simulink model "Benchmark2021ControllerNew"  (R2018a)
settings: Solver=ode1  StartTime=0  StopTime=t_end  FixedStep=simTs  RelTol=1e-3
values from neighbouring files (symbols this model uses):
  Horizon_Lowlayer = T_PreDomn-T_Apply    [Initial_Lower.m]
  Initial_headway = Sensor_FOL_dDist(2)    [Initial_main.m]
  Initial_MG1_spd = 0    [Initial_Lower.m]
  Initial_MG2_spd = 0    [Initial_Lower.m]
  Initial_SOC = 50    [Initial_main.m]
  Initial_vhcl_spd = 0    [Initial_main.m]
  N_opt = zeros(1,length(Power_ex))    [Initial_Lower.m]
  N_PMP_Lowlayer = Horizon_Lowlayer/Sampling_Lowlayer    [Initial_Lower.m]
  Power_level = 0:200:62800    [Initial_Lower.m]
  ras2rpm = 60/2/pi    (= 9.54929658551)    [Initial_main.m]
  Route_Destination_Distance = 16002    [Initial_Upper.m]
  rpm2rads = 1/rads2rpm    (= 0.10471975512)    [Initial_Lower.m]    (also in Initial_main.m)
  Sampling_Lowlayer = 0.05    [Initial_Lower.m]
  T_opt = zeros(1,length(Power_ex))    [Initial_Lower.m]
undefined symbols (not defined in the file or in its folder): DiscIntNeverNeededParam, Maxtorque_EngTrq, MG2_MaxMintorque_MaxTrq, MG2_MaxMintorque_Spd, Rc2, Rf1, Rf2, Rm, Rt, UpperLayerVpredict
(part 11 of 11)

== matlab function Benchmark2021ControllerNew/DesignController/Benchmark-Controller/Speed Prediction/MATLAB Function1 ==
  data: u input; y output
function y = fcn(u)

y = u(1:end-1);
